simulink model "A3_model_cc_prob_9"  (R2024a)
settings: Solver=ode45  StartTime=0.0  StopTime=70  MaxStep=1e-3  RelTol=1e-3
values from neighbouring files (symbols this model uses):
  A_f = data(7)    [A3_41.m]
  C_D = data(6)    [A3_41.m]
  f = data(8)    [A3_41.m]
  g = 9.82    [A3_41.m]
  k = data(2)    [A3_41.m]
  K_aug = [0.000079462857141, 2.571858424587528, 0.927433309066289]    [A3_41.m]
  m = data(1)    [A3_41.m]
  r_gear = data(4)    [A3_41.m]
  r_w = data(5)    [A3_41.m]
  rho = 1.2    [A3_41.m]
  tau = data(3)    [A3_41.m]
  u_e = 0.1448    [A3_41.m]
  x1_e = 2550    [A3_41.m]
  x2_e = 15    [A3_41.m]
settings Model: Creator=jofr  LastModifiedBy=munav
settings SolverCC: AlgebraicLoopSolver=TrustRegion
settings DataIOCC: LimitDataPoints=on  SaveFormat=Array  SignalLoggingSaveFormat=ModelDataLogs  ReturnWorkspaceOutputs=off
settings OptimizationCC: BlockReduction=off  BooleanDataType=off  LifeSpan=inf
settings DebuggingCC: SaveWithParameterizedLinksMsg=none  UnderspecifiedInitializationDetection=Classic  MergeDetectMultiDrivingBlocksExec=none  SignalResolutionControl=TryResolveAllWithWarning  MultiTaskDSMMsg=warning  MultiTaskCondExecSysMsg=none  UnconnectedInputMsg=warning  UnconnectedOutputMsg=warning  UnconnectedLineMsg=warning  SFUnexpectedBacktrackingDiag=warning  SFNoUnconditionalDefaultTransitionDiag=warning  SFExecutionAtInitializationDiag=none  ArithmeticOperatorsInVariantConditions=warning
settings HardwareCC: ProdBitPerPointer=32  ProdBitPerSizeT=32  ProdBitPerPtrDiffT=32  ProdLargestAtomicFloat=None  ProdIntDivRoundTo=Undefined  ProdEndianess=Unspecified  ProdWordSize=32  ProdHWDeviceType=32-bit Generic  TargetUnknown=on
settings ModelReferenceCC: EnableRefExpFcnMdlSchedulingChecks=on  PropagateSignalLabelsOutOfModel=off
settings SFSimCC: SimUseLocalCustomCode=off  CustomCodeUndefinedFunction=UseInterfaceOnly
settings RTWCC: RTWUseLocalCustomCode=off  GPUComputeCapability=3.5  DLArmComputeVersion=19.05
settings CodeAppCC: StateflowObjectComments=on
settings GRTTargetCC: TargetLangStandard=C89/C90 (ANSI)
settings ConfigComp: CovMetricSettings=dw  CovSaveCumulativeToWorkspaceVar=on  CovSaveSingleToWorkspaceVar=on  CovExternalEMLEnable=off

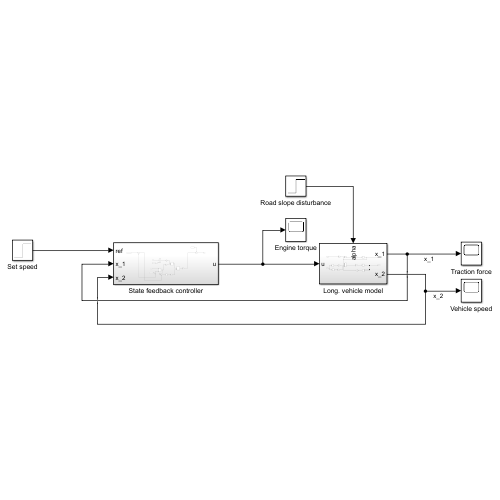
[thumbnail: Simulink's stored preview of the top-level diagram]
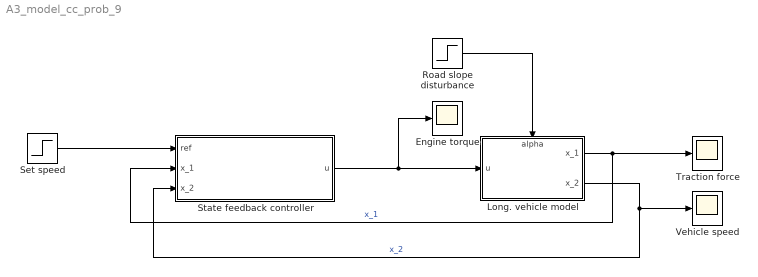
== system A3_model_cc_prob_9 ==
  Engine torque : Scope
  Long. vehicle model : Subsystem
      settings: PortSchema="{\"entries\":[{\"content\":{\"sides\":[{\"content\":{\"connectorIds\":[\"In1\"]},\"type\":\"ConnectorPlacement.EquallySpacedRectSide\",\"uuid\":\"51f5580e-5c6e-4005-9512-bdadc281ac3a\"},{\"content\":{\"connectorIds\":[\"Out1\",\"Out2\"],\"side\":\"RIGHT\"},\"type\":\"ConnectorPlacement.EquallySpacedRectSide\",\"uuid\":\"d841b77a-3407-4f39-8145-3c049402f25c\"},{\"content\":{\"connectorIds\":[\"In2\"],\"side\":\"TOP\"},\"type\":\"ConnectorPlacement.EquallySpacedRectSide\",\"uuid\":\"59296623-80a5-431d-9ae6-ee17199b70f7\"},{\"content\":{\"connectorIds\":[],\"side\":\"HIDDEN\"},\"type\":\"ConnectorPlacement.EquallySpacedRectSide\",\"uuid\":\"7f9b0e8e-917b-4707-8477-31ec1d3d2eee\"}]},\"type\":\"ConnectorPlacement.EquallySpacedConnector\",\"uuid\":\"993d3ed7-592f-4af3-96ae-7f032c513b4f\"}],\"packageUris\":[\"http://schema.mathworks.com/mf0/Connector/R2020b\"],\"version\":\"1.0\"}"
  Road slope disturbance : Step  Time=30  After=0.1  SampleTime=0
  Set speed : Step  Time=5  Before=15  After=20  SampleTime=0
  State feedback controller : Subsystem
  Traction force : Scope
  Vehicle speed : Scope
  wires:
  Long. vehicle model/1(x_1) -> Traction force/1, State feedback controller/2(x_1)  "x_1"
  Long. vehicle model/2(x_2) -> State feedback controller/3(x_2), Vehicle speed/1  "x_2"
  Road slope disturbance/1 -> Long. vehicle model/2(alpha)
  State feedback controller/1(u) -> Engine torque/1, Long. vehicle model/1(u)
  Set speed/1 -> State feedback controller/1(ref)

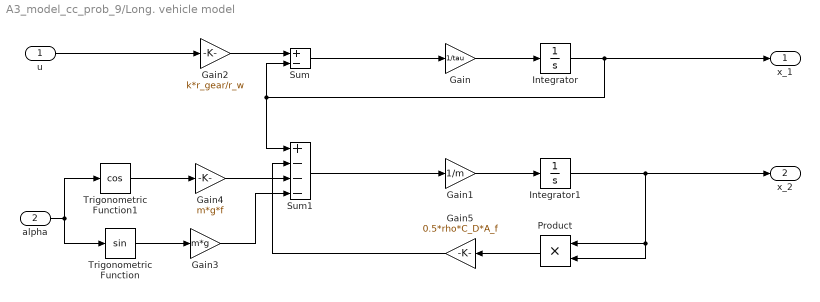
== system A3_model_cc_prob_9/Long. vehicle model ==
  u : Inport
  alpha : Inport  Port=2
  Gain : Gain  Gain=1/tau
  Gain1 : Gain  Gain=1/m
  Gain2 : Gain  Gain=k*r_gear/r_w
  Gain3 : Gain  Gain=m*g
  Gain4 : Gain  Gain=m*g*f
  Gain5 : Gain  Gain=0.5*rho*C_D*A_f
  Integrator : Integrator  InitialCondition=x1_e
  Integrator1 : Integrator  InitialCondition=x2_e
  Product : Product
  Sum : Sum  Inputs=+-
  Sum1 : Sum  Inputs=+---
  Trigonometric Function : Trigonometry
  Trigonometric Function1 : Trigonometry  Operator=cos
  x_1 : Outport
  x_2 : Outport  Port=2
  wires:
  Integrator/1 -> Sum/2, Sum1/1, x_1/1
  Gain/1 -> Integrator/1
  Gain1/1 -> Integrator1/1
  Sum1/1 -> Gain1/1
  Sum/1 -> Gain/1
  Gain2/1 -> Sum/1
  u/1 -> Gain2/1
  alpha/1 -> Trigonometric Function1/1, Trigonometric Function/1
  Trigonometric Function/1 -> Gain3/1
  Gain3/1 -> Sum1/4
  Gain4/1 -> Sum1/3
  Trigonometric Function1/1 -> Gain4/1
  Integrator1/1 -> Product/2, Product/1, x_2/1
  Product/1 -> Gain5/1
  Gain5/1 -> Sum1/2

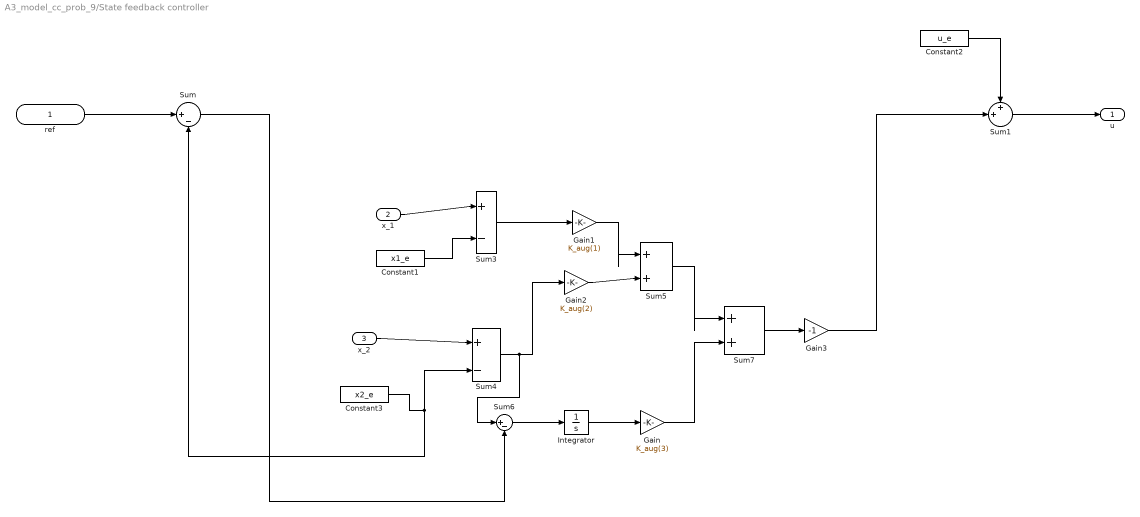
== system A3_model_cc_prob_9/State feedback controller ==
  ref : Inport
  x_1 : Inport  Port=2
  x_2 : Inport  Port=3
  Constant1 : Constant  Value=x1_e
  Constant2 : Constant  Value=u_e
  Constant3 : Constant  Value=x2_e
  Gain : Gain  Gain=K_aug(3)
  Gain1 : Gain  Gain=K_aug(1)
  Gain2 : Gain  Gain=K_aug(2)
  Gain3 : Gain  Gain=-1
  Integrator : Integrator
  Sum : Sum  Inputs=|+-
  Sum1 : Sum  Inputs=++|
  Sum3 : Sum  Inputs=|+|-
  Sum4 : Sum  Inputs=+|-
  Sum5 : Sum  Inputs=|++
  Sum6 : Sum  Inputs=|+-
  Sum7 : Sum  Inputs=|++
  u : Outport
  wires:
  Constant2/1 -> Sum1/1
  Sum1/1 -> u/1
  x_1/1 -> Sum3/1
  Constant1/1 -> Sum3/2
  x_2/1 -> Sum4/1
  Constant3/1 -> Sum4/2, Sum/2
  ref/1 -> Sum/1
  Sum3/1 -> Gain1/1
  Sum4/1 -> Sum6/1, Gain2/1
  Gain2/1 -> Sum5/2
  Gain1/1 -> Sum5/1
  Sum6/1 -> Integrator/1
  Integrator/1 -> Gain/1
  Sum5/1 -> Sum7/1
  Gain/1 -> Sum7/2
  Sum/1 -> Sum6/2
  Sum7/1 -> Gain3/1
  Gain3/1 -> Sum1/2
